simulink model "longitudinal_body"  (R2024b)
settings: Solver=VariableStepAuto  StartTime=0.0  StopTime=10  MaxStep=10^-3  RelTol=1e-5
undefined symbols (not defined in the file): car
libraries: autolibshared x1
settings Model: Creator=frank  LastModifiedBy=aless

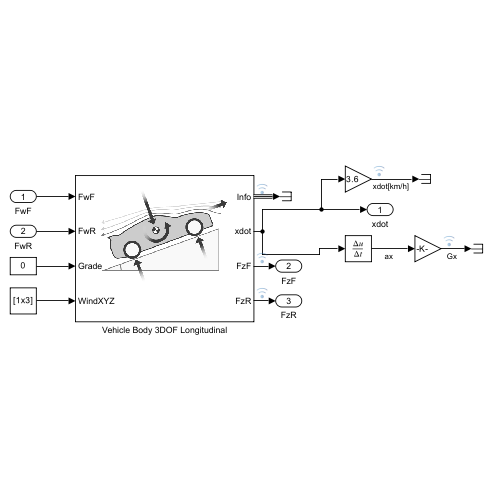
[thumbnail: Simulink's stored preview of the top-level diagram]
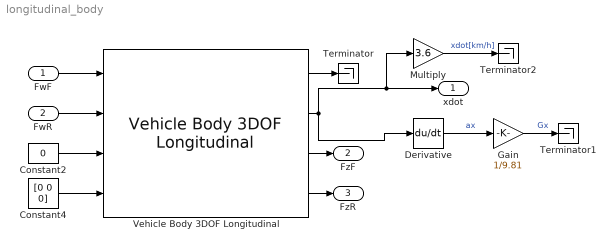
== system longitudinal_body ==
  FwF : Inport
  FwR : Inport  Port=2
  Constant2 : Constant  Value=0
  Constant4 : Constant  Value=[0 0 0]
  Derivative : Derivative
  Gain : Gain  Gain=1/9.81
  Multiply : Gain  Gain=3.6
  Terminator : Terminator
  Terminator1 : Terminator
  Terminator2 : Terminator
  Vehicle Body 3DOF Longitudinal : autolibshared/Vehicle Body 3DOF Longitudinal  VariantControl=SL  groundType=Grade angle  aMode=2  extFMode=off  extMMode=off  extTamb=off  NF=2  NR=2  m=car.Longitudinalbody.Mass  a=car.Longitudinalbody.COGa  b=car.Longitudinalbody.COGb  h=car.Longitudinalbody.COGh  Cd=car.Longitudinalbody.Cd  Af=car.Longitudinalbody.Af  x_o=0  xdot_o=0  Cl=car.Longitudinalbody.Cl  z_o=car.Longitudinalbody.COGz_o  zdot_o=0  Iyy=car.Longitudinalbody.I(2)  Cpm=.1  theta_o=0  q_o=0  FskF=car.Longitudinalbody.FskF  dzsF=car.Longitudinalbody.dzsF  FsbF=car.Longitudinalbody.FsbF  dzdotsF=car.Longitudinalbody.dzdotsF  FskR=car.Longitudinalbody.FskR  dzsR=car.Longitudinalbody.dzsR  FsbR=car.Longitudinalbody.FsbR  dzdotsR=car.Longitudinalbody.dzdotsR  Pabs=101325  T=273  g=9.81  blkID=0
      settings: LibrarySourceBlock=vehdynlibeom/Vehicle Body 3DOF Longitudinal
  xdot : Outport
  FzF : Outport  Port=2
  FzR : Outport  Port=3
  wires:
  Constant2/1 -> Vehicle Body 3DOF Longitudinal/3
  FwF/1 -> Vehicle Body 3DOF Longitudinal/1
  Vehicle Body 3DOF Longitudinal/4 -> FzR/1
  Vehicle Body 3DOF Longitudinal/2 -> Derivative/1, xdot/1, Multiply/1
  Vehicle Body 3DOF Longitudinal/3 -> FzF/1
  Constant4/1 -> Vehicle Body 3DOF Longitudinal/4
  Vehicle Body 3DOF Longitudinal/1 -> Terminator/1
  FwR/1 -> Vehicle Body 3DOF Longitudinal/2
  Derivative/1 -> Gain/1  "ax"
  Gain/1 -> Terminator1/1  "Gx"
  Multiply/1 -> Terminator2/1  "xdot[km/h]"
